simulink model "car_kine4"  (R2019a)
settings: Solver=VariableStepAuto  StartTime=0.0  StopTime=20.0  RelTol=1e-3
undefined symbols (not defined in the file or in its folder): cal_P
libraries: simulink x2
settings Model: Creator=mi  LastModifiedBy=mi

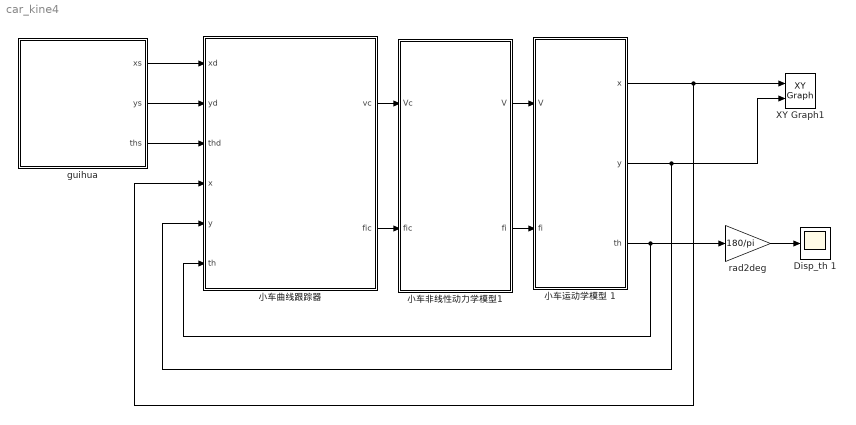
== system car_kine4 ==
  Disp_th 1 : Scope
  XY Graph1 : simulink/Sinks/XY Graph  xmin=-3  xmax=3  ymin=-0.2  ymax=5.2  st=-1
  "guihua " : Subsystem
  rad2deg : Gain  Gain=180/pi
  "小车曲线跟踪器 " : Subsystem
  小车运动学模型 1 : Subsystem  mask{L=0.254}
      mask prompts: L "小车车长L(米)"
  小车非线性动力学模型1 : Subsystem  mask{M=1.4175, L=0.254, W=6.5*2.54/100, bu=14.175, b=3.5*2.54/100, Tv=0.1, Tfi=0.1}
      mask prompts: M "小车质量(千克)"; L "车长(米)"; W "车宽(米)"; bu "小车前向阻尼系数"; b "小车质心到后轮的距离(米)"; Tv "小车速度驱动时间常数(秒)"; Tfi "小车转向驱动时间常数(秒)"
      mask init:
      | J=M*(L^2+W^2)/12
  wires:
  "guihua "/1("xs ") -> "小车曲线跟踪器 "/1(xd)
  "guihua "/2("ys ") -> "小车曲线跟踪器 "/2(yd)
  "guihua "/3("ths ") -> "小车曲线跟踪器 "/3(thd)
  "小车曲线跟踪器 "/1(vc) -> 小车非线性动力学模型1/1(Vc)
  "小车曲线跟踪器 "/2(fic) -> 小车非线性动力学模型1/2(fic)
  小车非线性动力学模型1/1(V) -> 小车运动学模型 1/1(V)
  小车非线性动力学模型1/2("fi ") -> 小车运动学模型 1/2(fi)
  小车运动学模型 1/1(x) -> XY Graph1/1, "小车曲线跟踪器 "/4(x)
  小车运动学模型 1/2(y) -> XY Graph1/2, "小车曲线跟踪器 "/5(y)
  rad2deg/1 -> Disp_th 1/1
  小车运动学模型 1/3("th ") -> rad2deg/1, "小车曲线跟踪器 "/6(th)

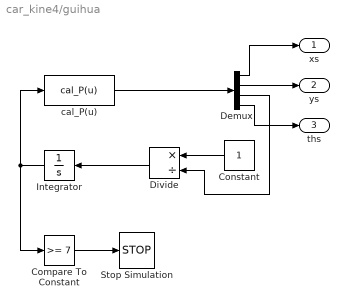
== system car_kine4/guihua  ==
  Compare To Constant : simulink/Logic and Bit Operations/Compare To Constant  relop=>=  const=7  OutDataTypeStr=boolean
  Constant : Constant
  Demux : Demux
  Divide : Product  Inputs=*/
  Integrator : Integrator
  Stop Simulation : Stop
  cal_P(u) : MATLABFcn  MATLABFcn=cal_P(u)  OutputDimensions=4
  "xs " : Outport
  "ys " : Outport  Port=2
  "ths " : Outport  Port=3
  wires:
  Constant/1 -> Divide/1
  Demux/3 -> Divide/2
  Integrator/1 -> Compare To Constant/1, cal_P(u)/1
  cal_P(u)/1 -> Demux/1
  Divide/1 -> Integrator/1
  Demux/2 -> "ys "/1
  Compare To Constant/1 -> Stop Simulation/1
  Demux/1 -> "xs "/1
  Demux/4 -> "ths "/1

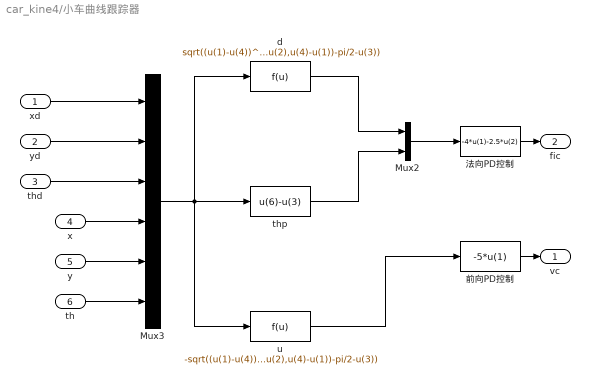
== system car_kine4/小车曲线跟踪器  ==
  xd : Inport
  yd : Inport  Port=2
  thd : Inport  Port=3
  x : Inport  Port=4
  y : Inport  Port=5
  th : Inport  Port=6
  Mux2 : Mux  Inputs=2
  Mux3 : Mux  Inputs=6
  d : Fcn  Expr=sqrt((u(1)-u(4))^2+(u(2)-u(5))^2)*cos(atan2(u(5)-u(2),u(4)-u(1))-pi/2-u(3))
  thp : Fcn  Expr=u(6)-u(3)
  u : Fcn  Expr=-sqrt((u(1)-u(4))^2+(u(2)-u(5))^2)*sin(atan2(u(5)-u(2),u(4)-u(1))-pi/2-u(3))
  前向PD控制 : Fcn  Expr=-5*u(1)
  法向PD控制 : Fcn  Expr=-4*u(1)-2.5*u(2)
  vc : Outport
  fic : Outport  Port=2
  wires:
  xd/1 -> Mux3/1
  u/1 -> 前向PD控制/1
  Mux3/1 -> u/1, d/1, thp/1
  x/1 -> Mux3/4
  Mux2/1 -> 法向PD控制/1
  thp/1 -> Mux2/2
  d/1 -> Mux2/1
  yd/1 -> Mux3/2
  th/1 -> Mux3/6
  前向PD控制/1 -> vc/1
  y/1 -> Mux3/5
  thd/1 -> Mux3/3
  法向PD控制/1 -> fic/1

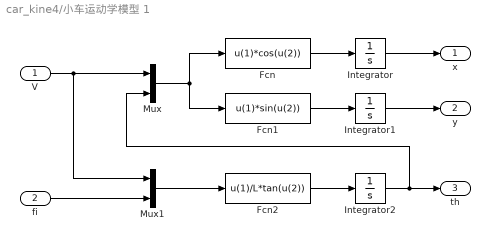
== system car_kine4/小车运动学模型 1 ==
  V : Inport
  fi : Inport  Port=2
  Fcn : Fcn  Expr=u(1)*cos(u(2))
  Fcn1 : Fcn  Expr=u(1)*sin(u(2))
  Fcn2 : Fcn  Expr=u(1)/L*tan(u(2))
  Integrator : Integrator
  Integrator1 : Integrator
  Integrator2 : Integrator
  Mux : Mux  Inputs=2
  Mux1 : Mux  Inputs=2
  x : Outport
  y : Outport  Port=2
  "th " : Outport  Port=3
  wires:
  Fcn1/1 -> Integrator1/1
  Integrator/1 -> x/1
  V/1 -> Mux/1, Mux1/1
  Mux/1 -> Fcn1/1, Fcn/1
  Integrator1/1 -> y/1
  fi/1 -> Mux1/2
  Fcn2/1 -> Integrator2/1
  Mux1/1 -> Fcn2/1
  Fcn/1 -> Integrator/1
  Integrator2/1 -> Mux/2, "th "/1

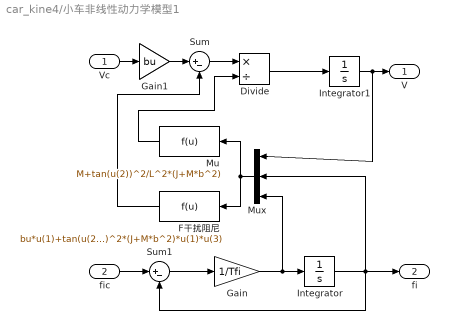
== system car_kine4/小车非线性动力学模型1 ==
  Vc : Inport
  fic : Inport  Port=2
  Divide : Product  Inputs=*/
  F干扰阻尼 : Fcn  Expr=bu*u(1)+tan(u(2))/L^2/cos(u(2))^2*(J+M*b^2)*u(1)*u(3)
  Gain : Gain  Gain=1/Tfi
  Gain1 : Gain  Gain=bu
  Integrator : Integrator
  Integrator1 : Integrator
  Mu : Fcn  Expr=M+tan(u(2))^2/L^2*(J+M*b^2)
  Mux : Mux  Inputs=3
  Sum : Sum  Inputs=|+-
  Sum1 : Sum  Inputs=|+-
  V : Outport
  "fi " : Outport  Port=2
  wires:
  Gain1/1 -> Sum/1
  Vc/1 -> Gain1/1
  F干扰阻尼/1 -> Sum/2
  Mu/1 -> Divide/2
  Mux/1 -> Mu/1, F干扰阻尼/1
  Sum/1 -> Divide/1
  Divide/1 -> Integrator1/1
  Integrator1/1 -> V/1, Mux/1
  Integrator/1 -> "fi "/1, Sum1/2, Mux/2
  Gain/1 -> Integrator/1, Mux/3
  Sum1/1 -> Gain/1
  fic/1 -> Sum1/1
